simulink library "Primary_Resistance_Start"  (R2024a)
settings: Solver=VariableStepAuto  StartTime=0.0  StopTime=10.0  RelTol=1e-3
libraries: spsBreakerLib x9, spsSeriesRLCBranchLib x9
settings Model: Creator=gshma  LastModifiedBy=gshma

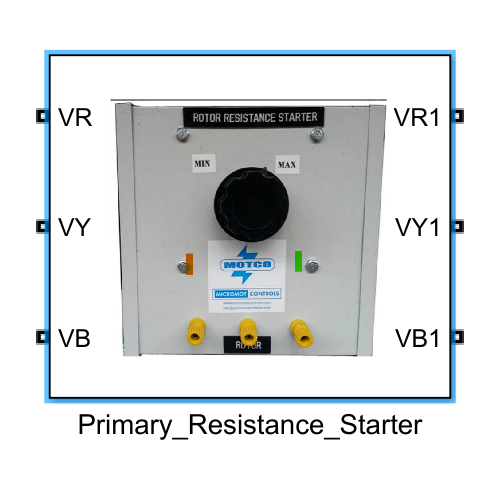
[thumbnail: Simulink's stored preview of the top-level diagram]
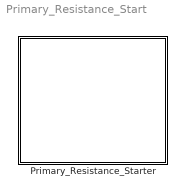
== system Primary_Resistance_Start ==
  Primary_Resistance_Starter : Subsystem
      mask Display: image('pems.png', [0,0,0,0,75,75]);

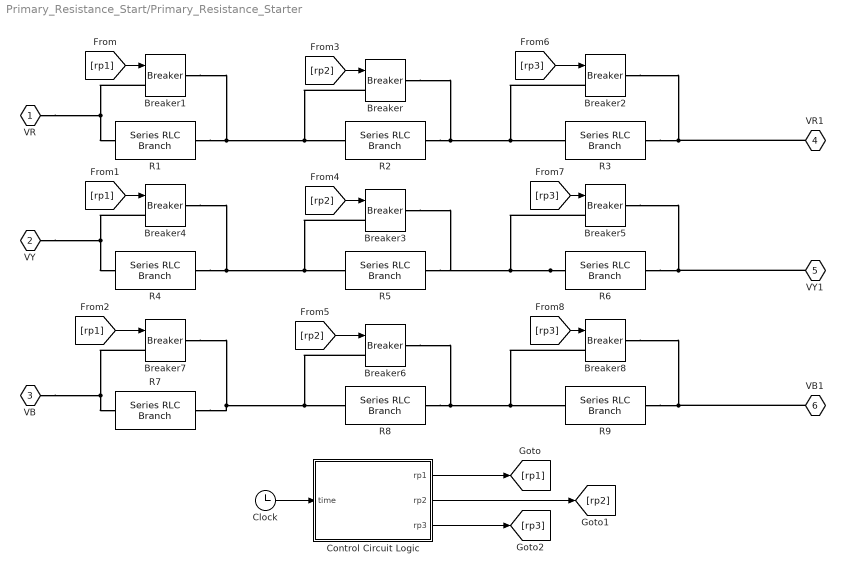
== system Primary_Resistance_Start/Primary_Resistance_Starter ==
  Breaker{,1..8} (9 alike) : spsBreakerLib/Breaker  InitialState=0  SwitchingTimes="[1/60  5/60]"  External=on  BreakerResistance=0.01  SnubberResistance=1e6  SnubberCapacitance=inf  Measurements=None  MoreParameters=on  NoBreakLoop=off
  Clock : Clock
  Control Circuit Logic : MATLAB Function  TreatAsAtomicUnit=on
  R1 : spsSeriesRLCBranchLib/Series RLC Branch  LConnTagsString=__new0  RConnTagsString=__new0  BranchType=R  Resistance=1  Inductance=1e-3  SetiL0=off  InitialCurrent=0  Capacitance=1e-6  Setx0=off  InitialVoltage=0  Measurements=None
  R2 : spsSeriesRLCBranchLib/Series RLC Branch  LConnTagsString=__new0  RConnTagsString=__new0  BranchType=R  Resistance=1.5  Inductance=1e-3  SetiL0=off  InitialCurrent=0  Capacitance=1e-6  Setx0=off  InitialVoltage=0  Measurements=None
  R3 : spsSeriesRLCBranchLib/Series RLC Branch  LConnTagsString=__new0  RConnTagsString=__new0  BranchType=R  Resistance=2.5  Inductance=1e-3  SetiL0=off  InitialCurrent=0  Capacitance=1e-6  Setx0=off  InitialVoltage=0  Measurements=None
  R4 : spsSeriesRLCBranchLib/Series RLC Branch  LConnTagsString=__new0  RConnTagsString=__new0  BranchType=R  Resistance=1  Inductance=1e-3  SetiL0=off  InitialCurrent=0  Capacitance=1e-6  Setx0=off  InitialVoltage=0  Measurements=None
  R5 : spsSeriesRLCBranchLib/Series RLC Branch  LConnTagsString=__new0  RConnTagsString=__new0  BranchType=R  Resistance=1.5  Inductance=1e-3  SetiL0=off  InitialCurrent=0  Capacitance=1e-6  Setx0=off  InitialVoltage=0  Measurements=None
  R6 : spsSeriesRLCBranchLib/Series RLC Branch  LConnTagsString=__new0  RConnTagsString=__new0  BranchType=R  Resistance=2.5  Inductance=1e-3  SetiL0=off  InitialCurrent=0  Capacitance=1e-6  Setx0=off  InitialVoltage=0  Measurements=None
  R7 : spsSeriesRLCBranchLib/Series RLC Branch  LConnTagsString=__new0  RConnTagsString=__new0  BranchType=R  Resistance=1  Inductance=1e-3  SetiL0=off  InitialCurrent=0  Capacitance=1e-6  Setx0=off  InitialVoltage=0  Measurements=None
  R8 : spsSeriesRLCBranchLib/Series RLC Branch  LConnTagsString=__new0  RConnTagsString=__new0  BranchType=R  Resistance=1.5  Inductance=1e-3  SetiL0=off  InitialCurrent=0  Capacitance=1e-6  Setx0=off  InitialVoltage=0  Measurements=None
  R9 : spsSeriesRLCBranchLib/Series RLC Branch  LConnTagsString=__new0  RConnTagsString=__new0  BranchType=R  Resistance=2.5  Inductance=1e-3  SetiL0=off  InitialCurrent=0  Capacitance=1e-6  Setx0=off  InitialVoltage=0  Measurements=None
  VR : PMIOPort  Tag=simrfV2util1/Connection Port  Side=Left
  VY : PMIOPort  Tag=simrfV2util1/Connection Port  Port=2  Side=Left
  VB : PMIOPort  Tag=simrfV2util1/Connection Port  Port=3  Side=Left
  VR1 : PMIOPort  Tag=simrfV2util1/Connection Port  Port=4  Side=Right
  VY1 : PMIOPort  Tag=simrfV2util1/Connection Port  Port=5  Side=Right
  VB1 : PMIOPort  Tag=simrfV2util1/Connection Port  Port=6  Side=Right
  wires:
  Control Circuit Logic/2(rp2) -> [rp2]
  Control Circuit Logic/1(rp1) -> [rp1]
  [rp1] -> Breaker7/1
  [rp2] -> Breaker3/1
  [rp1] -> Breaker4/1
  [rp3] -> Breaker2/1
  [rp3] -> Breaker5/1
  [rp2] -> Breaker/1
  [rp2] -> Breaker6/1
  Control Circuit Logic/3(rp3) -> [rp3]
  [rp3] -> Breaker8/1
  Clock/1 -> Control Circuit Logic/1(time)
  [rp1] -> Breaker1/1
  connections:
  Breaker7/LConn1 -- VB/RConn1 -- R7/RConn1
  R2/LConn1 -- Breaker/RConn1 -- Breaker2/LConn1 -- R3/RConn1
  R6/RConn1 -- Breaker5/LConn1 -- Breaker3/RConn1 -- R5/LConn1
  R9/LConn1 -- VB1/RConn1 -- Breaker8/RConn1
  R4/LConn1 -- Breaker4/RConn1 -- Breaker3/LConn1 -- R5/RConn1
  R7/LConn1 -- Breaker7/RConn1 -- Breaker6/LConn1 -- R8/RConn1
  R8/LConn1 -- Breaker6/RConn1 -- Breaker8/LConn1 -- R9/RConn1
  R1/LConn1 -- Breaker1/RConn1 -- Breaker/LConn1 -- R2/RConn1
  Breaker4/LConn1 -- VY/RConn1 -- R4/RConn1
  R6/LConn1 -- VY1/RConn1 -- Breaker5/RConn1
  Breaker1/LConn1 -- VR/RConn1 -- R1/RConn1
  R3/LConn1 -- VR1/RConn1 -- Breaker2/RConn1

== matlab function Primary_Resistance_Start/Primary_Resistance_Starter/Control Circuit Logic ==
  data: time input; rp1 output; rp2 output; rp3 output
function [rp1,rp2,rp3] = Control_Logic(time)
    if time<0.5
        rp1 = false;
        rp2 = false;
        rp3 = false;
    elseif time>=0.5 && time<0.7
        rp1 = false;
        rp2 = false;
        rp3 = true;
    elseif time>=0.7 && time<1.2
        rp1 = false;
        rp2 = true;
        rp3 = true;
    else
        rp1 = true;
        rp2 = true;
        rp3 = true;
    end
end
